simulink model "pendulum_sim"  (R2021b)
settings: Solver=VariableStepAuto  StartTime=0.0  StopTime=30  RelTol=1e-3
values from neighbouring files (symbols this model uses):
  A_n = A-B*k    [lab5_workspace.m]
  B = [0 ... (first row only)    [lab5_workspace.m]
  C = [1,0,0,0 ... (first row only)    [lab5_workspace.m]
  D = [0;0;0;0]    [lab5_workspace.m]
undefined symbols (not defined in the file or in its folder): k
settings Model: Creator=DSDLn  LastModifiedBy=DSDLn

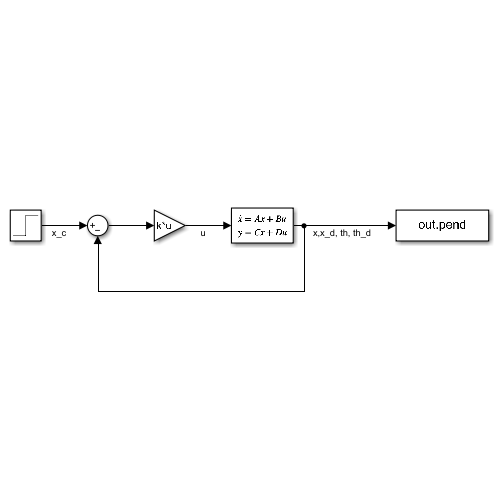
[thumbnail: Simulink's stored preview of the top-level diagram]
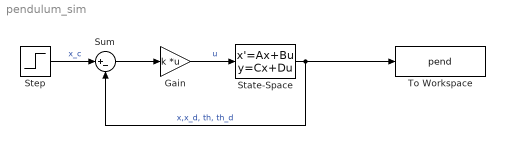
== system pendulum_sim ==
  Gain : Gain  Gain=k  Multiplication=Matrix(K*u)
  State-Space : StateSpace  A=A_n  B=B  C=C  D=D  InitialCondition=0
  Step : Step  Time=10  Before=[0;0;0;0]  After=[0.4;0;0;0]  SampleTime=0.01
  Sum : Sum  Inputs=|+-
  To Workspace : ToWorkspace  VariableName=pend  SampleTime=-1
  wires:
  Step/1 -> Sum/1  "x_c"
  Sum/1 -> Gain/1
  State-Space/1 -> To Workspace/1, Sum/2  "x,x_d, th, th_d"
  Gain/1 -> State-Space/1  "u"
